simulink model "Task6_1_a"  (Simulink 8.5)
settings: Solver=ode45  StartTime=0.0  StopTime=1000  RelTol=1e-3
libraries: simulink x1
settings Model: Creator=manso  LastModifiedBy=Quswar Mahmood Abid
settings DebuggingCC: SolverPrmCheckMsg=warning  FcnCallInpInsideContextMsg=UseLocalSettings

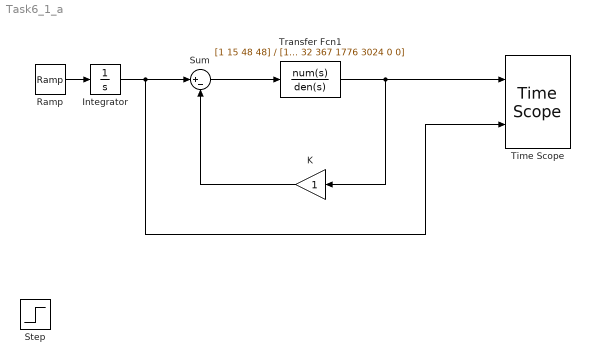
== system Task6_1_a ==
  Integrator : Integrator
  K : Gain
  Ramp : simulink/Sources/Ramp  slope=10  start=0  X0=0
  Step : Step  Time=0  After=5  SampleTime=0
  Sum : Sum  Inputs=|+-
  Time Scope : TimeScope  DefaultConfigurationName=spbscopes.TimeScopeBlockCfg  NumInputPorts=2
  Transfer Fcn1 : TransferFcn  Numerator=[1 15 48 48]  Denominator=[1 32 367 1776 3024 0 0]
  wires:
  Sum/1 -> Transfer Fcn1/1
  Transfer Fcn1/1 -> Time Scope/1, K/1
  K/1 -> Sum/2
  Ramp/1 -> Integrator/1
  Integrator/1 -> Sum/1, Time Scope/2
